simulink model "GUAM"  (R2024b)
settings: Solver=FixedStepAuto  StartTime=0.0  StopTime=SimIn.stopTime  FixedStep=SimIn.Environment.Turbulence.dT  RelTol=1e-6
values from neighbouring files (symbols this model uses):
  SimIn = setup(SimIn, userStruct.variants, target)    [simSetup.m]
undefined symbols (not defined in the file or in its folder): SimPar
libraries: dspnetwork x2, simulink x1, aerolibfltsims x1
settings Model: Creator=tbritton  LastModifiedBy=edison
settings SolverCC: AlgebraicLoopSolver=TrustRegion
settings DataIOCC: SaveFormat=Structure  SaveOutput=off  DSMLogging=off  SaveTime=off  ReturnWorkspaceOutputs=off
settings OptimizationCC: ReuseModelBlockBuffer=off
settings DebuggingCC: ReadBeforeWriteMsg=DisableAll  WriteAfterWriteMsg=DisableAll  WriteAfterReadMsg=DisableAll  MultiTaskDSMMsg=none  UnconnectedInputMsg=warning  UnconnectedOutputMsg=warning  UnconnectedLineMsg=warning  InitInArrayFormatMsg=none
settings ModelReferenceCC: UpdateModelReferenceTargets=IfOutOfDate  EnableRefExpFcnMdlSchedulingChecks=on
settings SFSimCC: SFSimEcho=off  CustomCodeUndefinedFunction=UseInterfaceOnly
settings RTWCC: GPUComputeCapability=3.5  DLArmComputeVersion=19.05

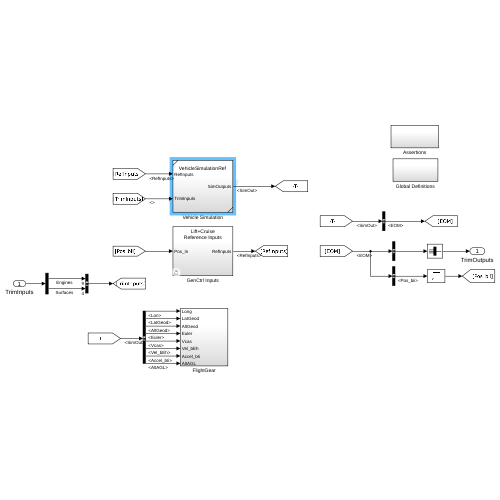
[thumbnail: Simulink's stored preview of the top-level diagram]
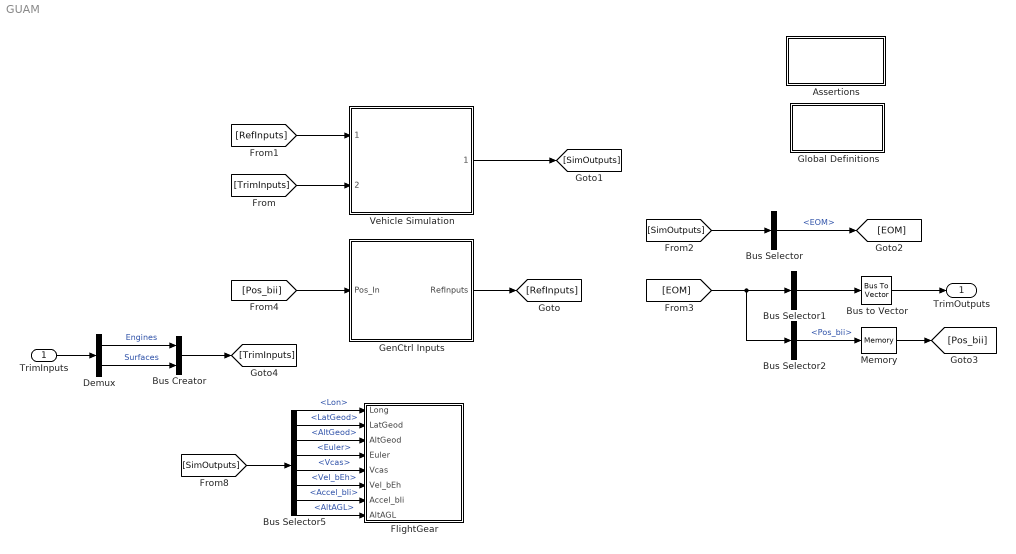
== system GUAM ==
  TrimInputs : Inport
  Assertions : Subsystem
  Bus Creator : BusCreator  Inputs=2  OutDataTypeStr=Bus: BUS_TRIM_INPUT
  Bus Selector : BusSelector  OutputSignals=Vehicle.EOM
  Bus Selector1 : BusSelector  OutputSignals=AirRelativeData.Veas,AirRelativeData.Vtot,AirRelativeData.alpha,AirRelativeData.beta,WorldRelativeData.gamma,WorldRelativeData.chi,InertialData.Asensed_bIb,AirRelativeData.Vtotdot,AirRelativeData.alphadot,AirRelativeData.betadot,WorldRelativeData.gammadot,WorldRelativeData.chidot,WorldRelativeData.VelDtH_bEh,WorldRelativeData.Euler.phi,WorldRelativeData.Euler.theta,WorldRelativeData.Euler.psi  OutputAsBus=on
  Bus Selector2 : BusSelector  OutputSignals=InertialData.Pos_bii
  Bus Selector5 : BusSelector  OutputSignals=Vehicle.EOM.WorldRelativeData.LatLonAlt.Lon,Vehicle.EOM.WorldRelativeData.LatLonAlt.LatGeod,Vehicle.EOM.WorldRelativeData.LatLonAlt.AltGeod,Vehicle.EOM.WorldRelativeData.Euler,Vehicle.EOM.AirRelativeData.Vcas,Vehicle.EOM.WorldRelativeData.Vel_bEh,Vehicle.EOM.InertialData.Accel_bIi,Vehicle.EOM.WorldRelativeData.AltAGL
  Bus to Vector : BusToVector
  Demux : Demux  Outputs=[SimIn.Trim.numEngines SimIn.Trim.numSurfaces]
  FlightGear : Subsystem
  GenCtrl Inputs : Subsystem  Variant=on  VariantControl=Variant1
  Global Definitions : Subsystem
  Memory : Memory
  Vehicle Simulation : Subsystem  ReferencedSubsystem=VehicleSimulationRef
  TrimOutputs : Outport  OutDataTypeStr=double  VectorParamsAs1DForOutWhenUnconnected=off
  wires:
  TrimInputs/1 -> Demux/1
  Bus to Vector/1 -> TrimOutputs/1
  Bus Selector1/1 -> Bus to Vector/1
  GenCtrl Inputs/1(RefInputs) -> [RefInputs]
  Vehicle Simulation/1 -> [SimOutputs]
  [TrimInputs] -> Vehicle Simulation/2
  [RefInputs] -> Vehicle Simulation/1
  [SimOutputs] -> Bus Selector/1
  Bus Selector/1 -> [EOM]  "<EOM>"
  Bus Creator/1 -> [TrimInputs]
  Demux/2 -> Bus Creator/2  "Surfaces"
  Demux/1 -> Bus Creator/1  "Engines"
  Bus Selector2/1 -> Memory/1  "<Pos_bii>"
  [EOM] -> Bus Selector1/1, Bus Selector2/1
  [Pos_bii] -> GenCtrl Inputs/1(Pos_In)
  Memory/1 -> [Pos_bii]
  Bus Selector5/8 -> FlightGear/8(AltAGL)  "<AltAGL>"
  Bus Selector5/7 -> FlightGear/7(Accel_bIi)  "<Accel_bIi>"
  Bus Selector5/6 -> FlightGear/6(Vel_bEh)  "<Vel_bEh>"
  Bus Selector5/5 -> FlightGear/5(Vcas)  "<Vcas>"
  Bus Selector5/4 -> FlightGear/4(Euler)  "<Euler>"
  Bus Selector5/3 -> FlightGear/3(AltGeod)  "<AltGeod>"
  Bus Selector5/2 -> FlightGear/2(LatGeod)  "<LatGeod>"
  Bus Selector5/1 -> FlightGear/1(Long)  "<Lon>"
  [SimOutputs] -> Bus Selector5/1

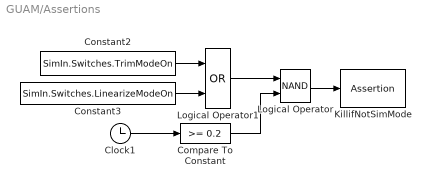
== system GUAM/Assertions ==
  Clock1 : Clock
  Compare To Constant : simulink/Logic and Bit Operations/Compare To Constant  relop=>=  const=0.2  OutDataTypeStr=boolean  ZeroCross=off
  Constant2 : Constant  Value=SimIn.Switches.TrimModeOn
  Constant3 : Constant  Value=SimIn.Switches.LinearizeModeOn
  KillifNotSimMode : Assertion  AssertionFailFcn="warndlg('Running simulation with TrimMode or LinearizeMode engaged.  Run setup.m to reset.','Warning!')"
  Logical Operator : Logic  Operator=NAND  AllPortsSameDT=off  OutDataTypeStr=boolean
  Logical Operator1 : Logic  Operator=OR  AllPortsSameDT=off  OutDataTypeStr=boolean
  wires:
  Constant2/1 -> Logical Operator1/1
  Compare To Constant/1 -> Logical Operator/2
  Clock1/1 -> Compare To Constant/1
  Logical Operator/1 -> KillifNotSimMode/1
  Constant3/1 -> Logical Operator1/2
  Logical Operator1/1 -> Logical Operator/1

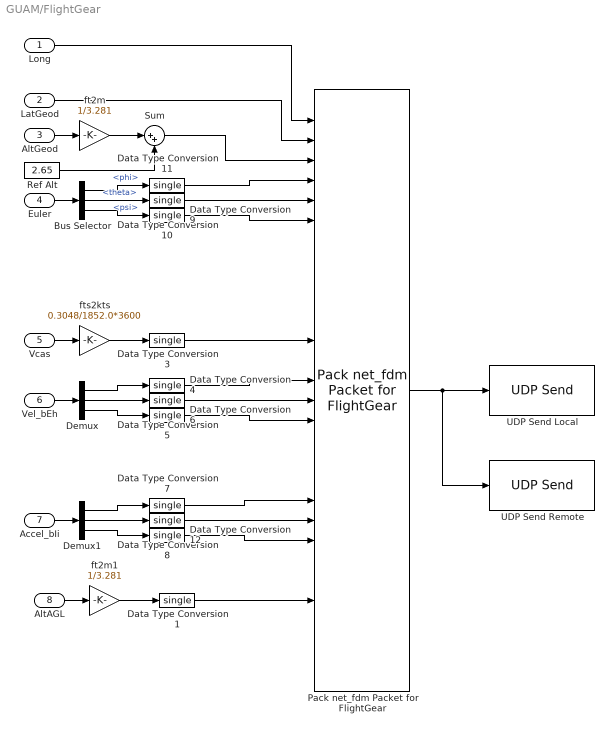
== system GUAM/FlightGear ==
  Long : Inport
  LatGeod : Inport  Port=2
  AltGeod : Inport  Port=3
  Euler : Inport  Port=4
  Vcas : Inport  Port=5
  Vel_bEh : Inport  Port=6
  Accel_bIi : Inport  Port=7
  AltAGL : Inport  Port=8
  Bus Selector : BusSelector  OutputSignals=phi,theta,psi
  Data Type Conversion{1,3..12} (11 alike) : DataTypeConversion  OutDataTypeStr=single  SaturateOnIntegerOverflow=off  RndMeth=Floor
  Demux : Demux  Outputs=3
  Demux1 : Demux  Outputs=3
  Pack net_fdm Packet for FlightGear : aerolibfltsims/Pack net_fdm Packet for FlightGear  FlightGearVersion=v2.4  ShowPositionAttitudeInputs=on  ShowVelocityAccelerationInputs=on  ShowControlSurfacePositionInputs=off  ShowEngineFuelInputs=off  ShowLandingGearInputs=off  ShowEnvironmentInputs=on  SampleTime=-1  packetVersion=24
  Ref Alt : Constant  Value=2.65
  Sum : Sum  Inputs=|++
  UDP Send Local : dspnetwork/UDP Send  remoteURL='127.0.0.1'  remotePort=simPortInput  localURL='0.0.0.0'  localPortSource=Automatically determine  localPort=-1  sendBufferSize=408  sampletime=-1  blockPlatform=[]  separateLengthPort=0
      settings: LibrarySourceBlock=dspsnks4/UDP Send
  UDP Send Remote : dspnetwork/UDP Send  remoteURL=simAddress  remotePort=simPortInput  localURL='0.0.0.0'  localPortSource=Automatically determine  localPort=-1  sendBufferSize=408  sampletime=-1  blockPlatform=[]  separateLengthPort=0
      settings: LibrarySourceBlock=dspsnks4/UDP Send
  ft2m : Gain  Gain=1/3.281
  ft2m1 : Gain  Gain=1/3.281
  fts2kts : Gain  Gain=0.3048/1852.0*3600
  wires:
  Pack net_fdm Packet for FlightGear/1 -> UDP Send Remote/1, UDP Send Local/1
  Ref Alt/1 -> Sum/2
  Sum/1 -> Pack net_fdm Packet for FlightGear/3
  Data Type Conversion1/1 -> Pack net_fdm Packet for FlightGear/25
  ft2m1/1 -> Data Type Conversion1/1
  AltAGL/1 -> ft2m1/1
  Bus Selector/3 -> Data Type Conversion9/1  "<psi>"
  Bus Selector/2 -> Data Type Conversion10/1  "<theta>"
  Bus Selector/1 -> Data Type Conversion11/1  "<phi>"
  Euler/1 -> Bus Selector/1
  Accel_bIi/1 -> Demux1/1
  Vel_bEh/1 -> Demux/1
  Vcas/1 -> fts2kts/1
  AltGeod/1 -> ft2m/1
  LatGeod/1 -> Pack net_fdm Packet for FlightGear/2
  Long/1 -> Pack net_fdm Packet for FlightGear/1
  fts2kts/1 -> Data Type Conversion3/1
  Data Type Conversion12/1 -> Pack net_fdm Packet for FlightGear/22
  Data Type Conversion8/1 -> Pack net_fdm Packet for FlightGear/21
  Data Type Conversion7/1 -> Pack net_fdm Packet for FlightGear/20
  Data Type Conversion6/1 -> Pack net_fdm Packet for FlightGear/16
  Data Type Conversion5/1 -> Pack net_fdm Packet for FlightGear/15
  Data Type Conversion4/1 -> Pack net_fdm Packet for FlightGear/14
  Demux1/3 -> Data Type Conversion12/1
  Demux1/2 -> Data Type Conversion8/1
  Demux1/1 -> Data Type Conversion7/1
  Demux/1 -> Data Type Conversion4/1
  Demux/2 -> Data Type Conversion5/1
  Demux/3 -> Data Type Conversion6/1
  ft2m/1 -> Sum/1
  Data Type Conversion3/1 -> Pack net_fdm Packet for FlightGear/12
  Data Type Conversion11/1 -> Pack net_fdm Packet for FlightGear/4
  Data Type Conversion10/1 -> Pack net_fdm Packet for FlightGear/5
  Data Type Conversion9/1 -> Pack net_fdm Packet for FlightGear/6

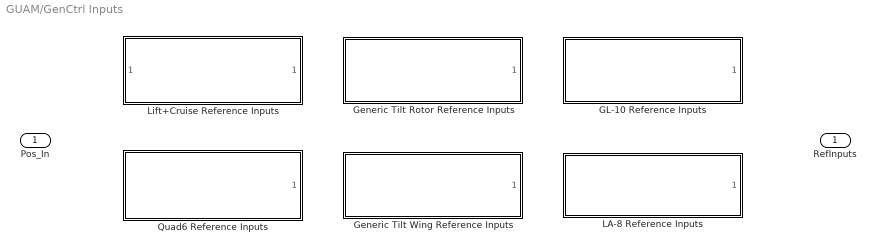
== system GUAM/GenCtrl Inputs ==
  Pos_In : Inport
  GL-10 Reference Inputs : Subsystem  VariantControl=GVS_VEH_TYPE_GL10  ReferencedSubsystem=GL_10_Reference_Inputs
  Generic Tilt Rotor Reference Inputs : Subsystem  VariantControl=GVS_VEH_TYPE_GTR  ReferencedSubsystem=GTR_Reference_Inputs
  Generic Tilt Wing Reference Inputs : Subsystem  VariantControl=GVS_VEH_TYPE_GTW  ReferencedSubsystem=GTW_Reference_Inputs
  LA-8 Reference Inputs : Subsystem  VariantControl=GVS_VEH_TYPE_LA8  ReferencedSubsystem=LA_8_Reference_Inputs
  Lift+Cruise Reference Inputs : Subsystem  VariantControl=GVS_VEH_TYPE_LC  ReferencedSubsystem=Lift_Cruise_Reference_Inputs
  Quad6 Reference Inputs : Subsystem  VariantControl=GVS_VEH_TYPE_QUAD6  ReferencedSubsystem=Quad6_Reference_Inputs
  RefInputs : Outport  OutDataTypeStr=Bus: BUS_REF_INPUT

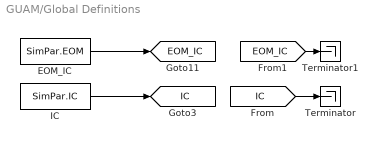
== system GUAM/Global Definitions ==
  EOM_IC : Constant  Value=SimPar.EOM  OutDataTypeStr=Bus: BUS_PARAM_EOM
  IC : Constant  Value=SimPar.IC  OutDataTypeStr=Bus: BUS_PARAM_IC
  Terminator : Terminator
  Terminator1 : Terminator
  tag scope: EOM_IC=global, IC=global
  wires:
  IC/1 -> [IC]
  EOM_IC/1 -> [EOM_IC]
  [IC] -> Terminator/1
  [EOM_IC] -> Terminator1/1
